simulink model "Scheme1"  (R2014a)
settings: Solver=VariableStepAuto  StartTime=0.0  StopTime=8  MaxStep=0.001  MinStep=0.0001  RelTol=1e-3
libraries: simulink x1
settings Model: Creator=hohotulca  LastModifiedBy=Анастасия
settings DataIOCC: SaveFormat=Dataset
settings OptimizationCC: SimCompilerOptimization=off
settings DebuggingCC: MergeDetectMultiDrivingBlocksExec=error  SolverPrmCheckMsg=none  FrameProcessingCompatibilityMsg=error  AllowSymbolicDim=off
settings HardwareCC: ProdBitPerPointer=64  ProdLargestAtomicFloat=Float  ProdIntDivRoundTo=Zero  ProdEndianess=LittleEndian  ProdWordSize=64  ProdHWDeviceType=Intel->x86-64 (Windows64)
settings RTWCC: RTWCompilerOptimization=off
settings GRTTargetCC: GeneratePreprocessorConditionals=Use local settings
settings ConfigComp: CovMetricSettings=dw  CovHtmlReporting=on  CovSaveCumulativeToWorkspaceVar=on  CovSaveSingleToWorkspaceVar=on  CovExternalEMLEnable=off

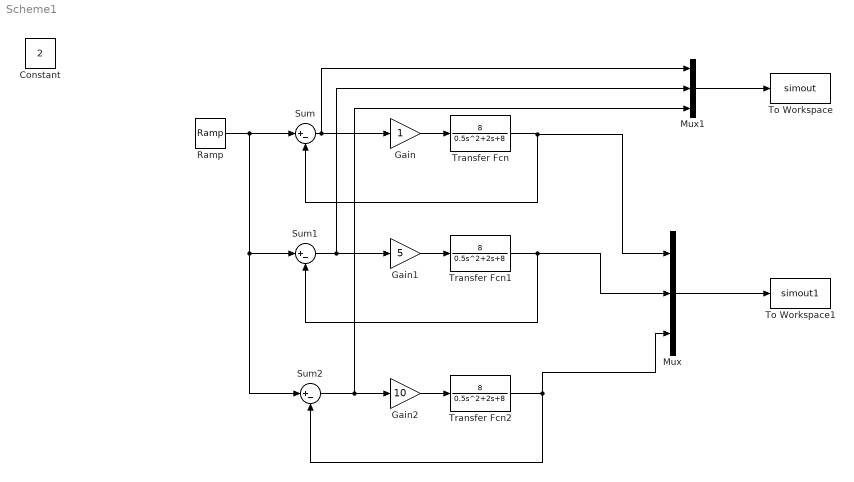
== system Scheme1 ==
  Constant : Constant  Value=2
  Gain : Gain
  Gain1 : Gain  Gain=5
  Gain2 : Gain  Gain=10
  Mux : Mux  Inputs=3
  Mux1 : Mux  Inputs=3
  Ramp : simulink/Sources/Ramp  slope=1  start=0  X0=0
  Sum : Sum  Inputs=|+-
  Sum1 : Sum  Inputs=|+-
  Sum2 : Sum  Inputs=|+-
  To Workspace : ToWorkspace  VariableName=simout  SaveFormat=Timeseries  SampleTime=-1
  To Workspace1 : ToWorkspace  VariableName=simout1  SaveFormat=Timeseries  SampleTime=-1
  Transfer Fcn : TransferFcn  Numerator=[8]  Denominator=[0.5 2 8]
  Transfer Fcn1 : TransferFcn  Numerator=[8]  Denominator=[0.5 2 8]
  Transfer Fcn2 : TransferFcn  Numerator=[8]  Denominator=[0.5 2 8]
  wires:
  Gain/1 -> Transfer Fcn/1
  Transfer Fcn/1 -> Mux/1, Sum/2
  Gain1/1 -> Transfer Fcn1/1
  Transfer Fcn1/1 -> Sum1/2, Mux/2
  Sum1/1 -> Mux1/2, Gain1/1
  Gain2/1 -> Transfer Fcn2/1
  Transfer Fcn2/1 -> Mux/3, Sum2/2
  Sum2/1 -> Gain2/1, Mux1/3
  Mux/1 -> To Workspace1/1
  Sum/1 -> Gain/1, Mux1/1
  Mux1/1 -> To Workspace/1
  Ramp/1 -> Sum2/1, Sum1/1, Sum/1
